simulink model "system"  (Simulink 7.5)
settings: Solver=ode3  StartTime=0.0  StopTime=10.0  RelTol=1e-3
settings Model: Creator=Josef  LastModifiedBy=Josef
settings DataIOCC: SaveFormat=StructureWithTime
settings OptimizationCC: ExpressionDepthLimit=128
settings DebuggingCC: UnderspecifiedInitializationDetection=Simplified  MergeDetectMultiDrivingBlocksExec=error  SolverPrmCheckMsg=none  FcnCallInpInsideContextMsg=Enable All  StateNameClashWarn=none
settings HardwareCC: ProdIntDivRoundTo=Zero  ProdEndianess=LittleEndian  ProdHWDeviceType=Intel->x86-32 (Windows32)
settings CodeAppCC: CustomSymbolStrType=$N$R$M_T
settings GRTTargetCC: TargetFunctionLibrary=C89/C90 (ANSI)  GeneratePreprocessorConditionals=Use local settings

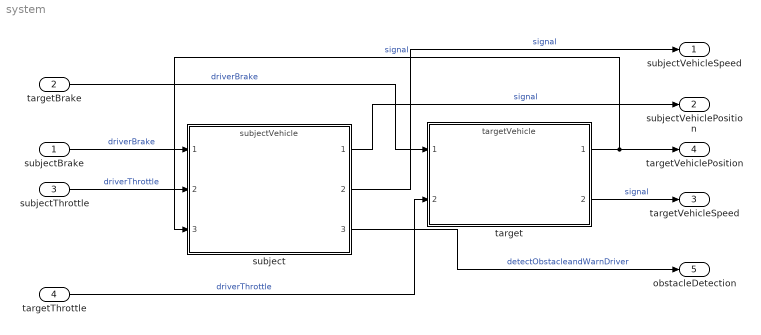
== system system ==
  subjectBrake : Inport
      settings: AttributesFormatString=driverBrake
  targetBrake : Inport  Port=2
      settings: AttributesFormatString=driverBrake
  subjectThrottle : Inport  Port=3
      settings: AttributesFormatString=driverThrottle
  targetThrottle : Inport  Port=4
      settings: AttributesFormatString=driverThrottle
  subject : ModelReference  ModelNameDialog=subjectVehicle  SimulationMode=Normal  ModelReferenceVersion=1.88  CopyOfModelName=subjectVehicle
  target : ModelReference  ModelNameDialog=targetVehicle  SimulationMode=Normal  ModelReferenceVersion=1.11  CopyOfModelName=subjectVehicle
  subjectVehicleSpeed : Outport
      settings: AttributesFormatString=signal
  subjectVehiclePosition : Outport  Port=2
      settings: AttributesFormatString=signal
  targetVehicleSpeed : Outport  Port=3
      settings: AttributesFormatString=signal
  targetVehiclePosition : Outport  Port=4
      settings: AttributesFormatString=signal
  obstacleDetection : Outport  Port=5
      settings: AttributesFormatString=detectObstacleandWarnDriver
  wires:
  target/1 -> subject/3, targetVehiclePosition/1  "signal"
  subjectBrake/1 -> subject/1  "driverBrake"
  targetBrake/1 -> target/1  "driverBrake"
  subjectThrottle/1 -> subject/2  "driverThrottle"
  targetThrottle/1 -> target/2  "driverThrottle"
  subject/1 -> subjectVehiclePosition/1  "signal"
  subject/2 -> subjectVehicleSpeed/1  "signal"
  target/2 -> targetVehicleSpeed/1  "signal"
  subject/3 -> obstacleDetection/1  "detectObstacleandWarnDriver"
